simulink model "post_lab_exercise"  (R2021b)
settings: Solver=VariableStepAuto  StartTime=0.0  StopTime=5  RelTol=1e-3
libraries: dspsrcs4 x3, dsparch4 x1
settings Model: Creator=Joshua  LastModifiedBy=Joshua

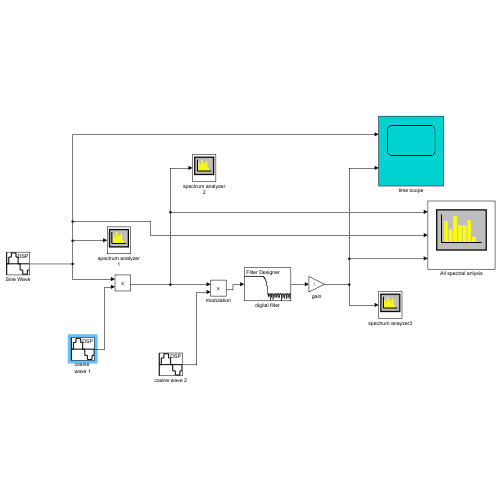
[thumbnail: Simulink's stored preview of the top-level diagram]
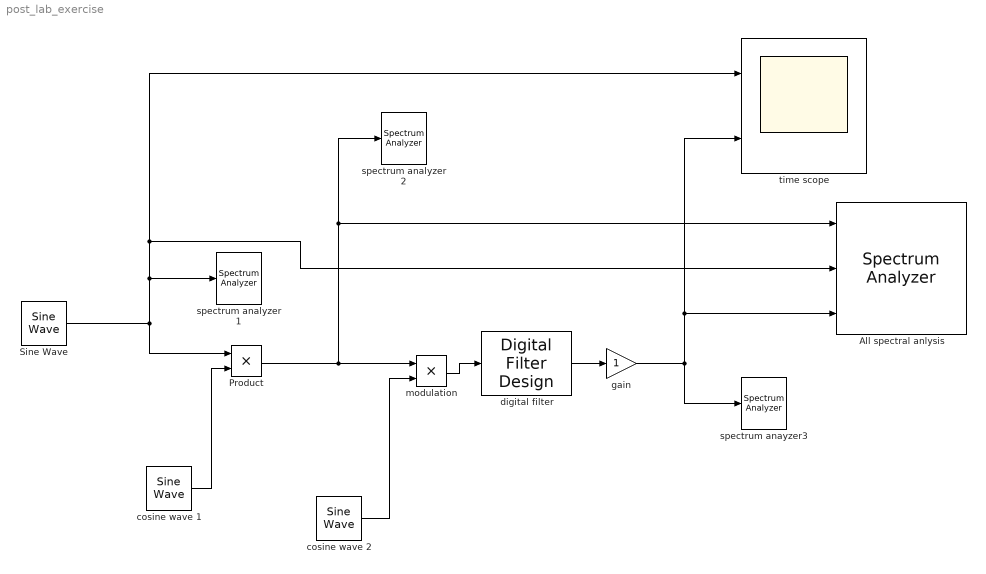
== system post_lab_exercise ==
  All spectral anlysis : SpectrumAnalyzer  NumInputPorts=3
  Product : Product
  Sine Wave : dspsrcs4/Sine Wave  Amplitude=1  Frequency=100  Phase=0  SampleMode=Discrete  OutComplex=Real  CompMethod=Trigonometric fcn  TableSize=Speed  SampleTime=1/1000  SamplesPerFrame=1  ResetState=Restart at time zero  OutputFrames=off  dataType=double  wordLen=16  udDataType=sfix(16)  fracBitsMode=Best precision  numFracBits=15  OutDataTypeStr=double  LastOutDataTypeStr=double
  cosine wave 1 : dspsrcs4/Sine Wave  Amplitude=1  Frequency=100  Phase=pi/2  SampleMode=Discrete  OutComplex=Real  CompMethod=Trigonometric fcn  TableSize=Speed  SampleTime=1/1000  SamplesPerFrame=1  ResetState=Restart at time zero  OutputFrames=off  dataType=double  wordLen=16  udDataType=sfix(16)  fracBitsMode=Best precision  numFracBits=15  OutDataTypeStr=double  LastOutDataTypeStr=double
  cosine wave 2 : dspsrcs4/Sine Wave  Amplitude=1  Frequency=100  Phase=pi/2  SampleMode=Discrete  OutComplex=Real  CompMethod=Trigonometric fcn  TableSize=Speed  SampleTime=1/1000  SamplesPerFrame=1  ResetState=Restart at time zero  OutputFrames=off  dataType=double  wordLen=16  udDataType=sfix(16)  fracBitsMode=Best precision  numFracBits=15  OutDataTypeStr=double  LastOutDataTypeStr=double
  digital filter : dsparch4/Digital Filter Design  mwdsp_browser_bugfix_var=off
  gain : Gain
  modulation : Product
  spectrum analyzer 1 : SpectrumAnalyzer
  spectrum analyzer 2 : SpectrumAnalyzer
  spectrum anayzer3 : SpectrumAnalyzer
  time scope : Scope  NumInputPorts=2
  wires:
  cosine wave 1/1 -> Product/2
  Sine Wave/1 -> All spectral anlysis/2, time scope/1, spectrum analyzer 1/1, Product/1
  cosine wave 2/1 -> modulation/2
  Product/1 -> spectrum analyzer 2/1, All spectral anlysis/1, modulation/1
  modulation/1 -> digital filter/1
  digital filter/1 -> gain/1
  gain/1 -> All spectral anlysis/3, time scope/2, spectrum anayzer3/1
